simulink model "borth"  (Simulink 6.4)
settings: Solver=FixedStepDiscrete  StartTime=0.0  StopTime=inf  RelTol=1e-3
undefined symbols (not defined in the file or in its folder): i
libraries: commsink2 x2, commdigbbndam3 x2, commchan3 x1, commrandsrc2 x1
settings Model: Creator=ALEX  LastModifiedBy=student
settings OptimizationCC: InitFltsAndDblsToZero=off
settings DebuggingCC: SignalResolutionControl=UseLocalSettings  MultiTaskDSMMsg=error  MultiTaskCondExecSysMsg=error
settings GRTTargetCC: TargetFcnLib=ansi_tfl_table_tmw.mat

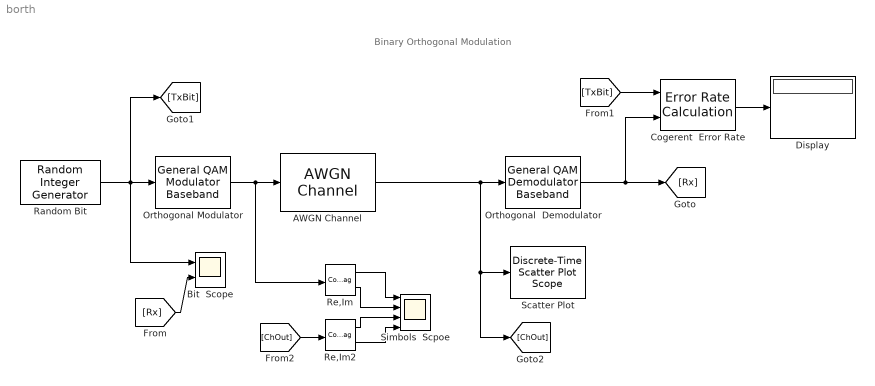
== system borth ==
  note: Binary Orthogonal Modulation
  AWGN Channel : commchan3/AWGN Channel  SystemSampleTime=-1  seed=67  noiseMode="Signal to noise ratio  (Es/No)"  EbNodB=3  EsNodB=100  SNRdB=10  bitsPerSym=1  Ps=1  Tsym=1  variance=0.2
  "Bit  Scope " : Scope  NumInputPorts=2
      settings: YMin=0~0  YMax=1.2~1.2
  Cogerent  Error Rate : commsink2/Error Rate Calculation  N=0  st_delay=0  cp_mode=Entire frame  subframe=[]  PMode=Port  WsName=ErrorVec  RsMode2=off  stop=off  numErr=100  maxBits=100000
  Display : Display
  Orthogonal Modulator : commdigbbndam3/General QAM Modulator Baseband  SigCon=[exp(pi*i*[0:1]/2)]*exp(i*pi*0/4)  outDtype=double  outWordLen=16  outUDDataType=sfix(16)  outFracLenMode=Best precision  outFracLen=15
  Orthogonal  Demodulator : commdigbbndam3/General QAM Demodulator Baseband  SigCon=[exp(pi*i*[0:1]/2)]  outDtype=int8
  Random Bit : commrandsrc2/Random Integer Generator  SystemSampleTime=-1  mul=2  seed=255  Ts=1  frameBased=off  sampPerFrame=8  orient=off  outDataType=int8
  Re,Im : ComplexToRealImag
  Re,Im2 : ComplexToRealImag
  Scatter Plot : commsink2/Discrete-Time Scatter Plot Scope  Tag=ScatterPlot  SystemSampleTime=-1  sampPerSymb=1  offsetEye=0  numTraces=100  numNewFrames=10  LineMarkers=.  LineColors=b  fading=on  render=on  AxisGrid=on  xMin=-2  xMax=2  yMin=-2  yMax=2  inphaseLabel=In-phase Amplitude  quadratureLabel=Quadrature Amplitude  openScopeAtSimStart=off  FrameNumber=off  FigPos=[360 362 560 560]  figTitle=Scatter Plot  numLinesMax=8  block_type_=scatter
  Simbols  Scpoe : Scope  NumInputPorts=4
      settings: YMin=0~0~0~0  YMax=1.2~1.2~1.2~1.2
  wires:
  AWGN Channel/1 -> Orthogonal  Demodulator/1, [ChOut], Scatter Plot/1
  Orthogonal  Demodulator/1 -> Cogerent  Error Rate/2, [Rx]
  Cogerent  Error Rate/1 -> Display/1
  Random Bit/1 -> "Bit  Scope "/1, Orthogonal Modulator/1, [TxBit]
  Orthogonal Modulator/1 -> AWGN Channel/1, Re,Im/1
  [Rx] -> "Bit  Scope "/2
  Re,Im/1 -> Simbols  Scpoe/1
  Re,Im/2 -> Simbols  Scpoe/2
  [TxBit] -> Cogerent  Error Rate/1
  Re,Im2/1 -> Simbols  Scpoe/3
  Re,Im2/2 -> Simbols  Scpoe/4
  [ChOut] -> Re,Im2/1
